simulink model "Motor_Model"  (Simulink 8.4)
settings: Solver=ode45  StartTime=0.0  StopTime=1  RelTol=1e-3
values from neighbouring files (symbols this model uses):
  eta = 0.9    [gs.m]
  g = 9.82    [gs.m]
  Ik = 0.004    [gs.m]
  Is = Ms*rs^2/2    (= 0.0005625)    [gs.m]
  J = 138E-7    (= 1.38e-05)    [gs.m]
  K_emf = 1/158    (= 0.00632911392405)    [gs.m]
  Kt = 60.3*10^-3    (= 0.0603)    [gs.m]
  l = 0.17    [gs.m]
  L = 0.329E-3    (= 0.000329)    [gs.m]
  max_current = 1    [gs.m]
  max_voltage = 48    [gs.m]
  Mtot = alu_mass + motor_mass + motor_power + arduino_mass + extra + M_s    (= 1.55)    [gs.m]
  Rm = 1.16    [gs.m]
settings Model: Creator=maen  LastModifiedBy=MikaelSjostedt
settings DataIOCC: LimitDataPoints=off

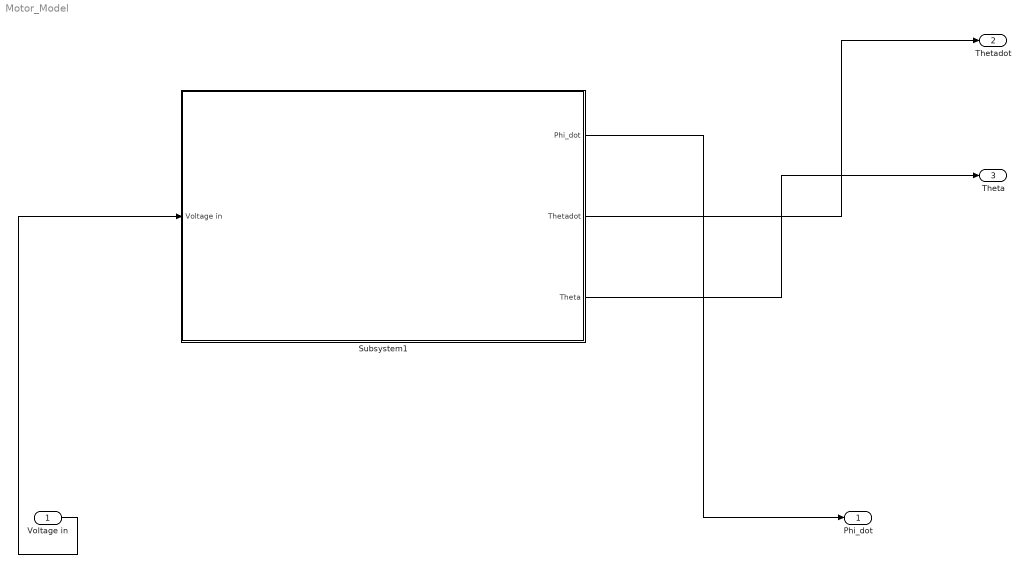
== system Motor_Model ==
  "Voltage in " : Inport
  Subsystem1 : Subsystem
  Phi_dot : Outport
  "Thetadot " : Outport  Port=2
  Theta : Outport  Port=3
  wires:
  "Voltage in "/1 -> Subsystem1/1("Voltage in ")
  Subsystem1/1(Phi_dot) -> Phi_dot/1
  Subsystem1/2("Thetadot ") -> "Thetadot "/1
  Subsystem1/3(Theta) -> Theta/1

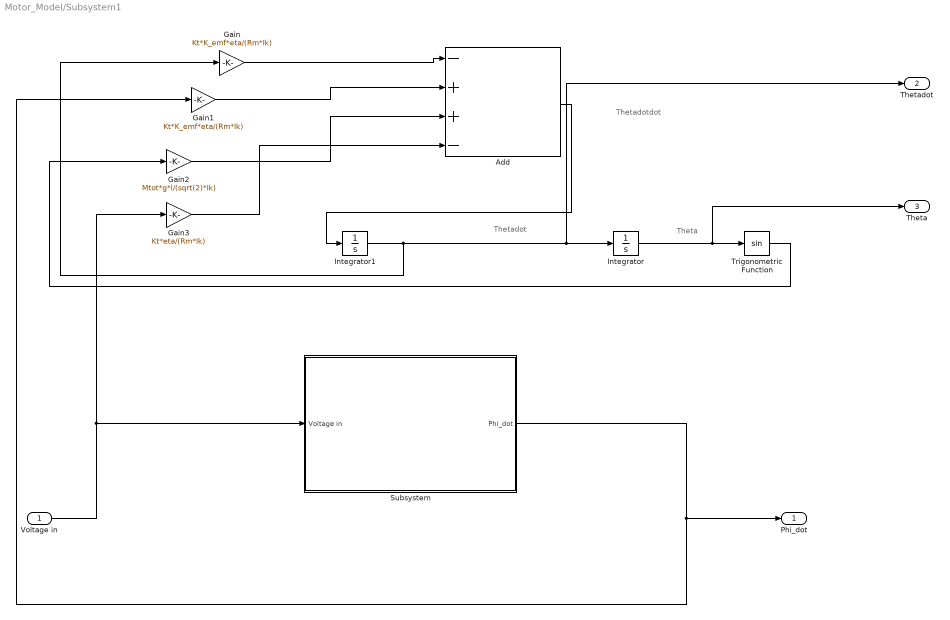
== system Motor_Model/Subsystem1 ==
  note: Theta
  note: Thetadot
  note: Thetadotdot
  "Voltage in " : Inport
  Add : Sum  Inputs=-++-
  Gain : Gain  Gain=Kt*K_emf*eta/(Rm*Ik)
  Gain1 : Gain  Gain=Kt*K_emf*eta/(Rm*Ik)
  Gain2 : Gain  Gain=Mtot*g*l/(sqrt(2)*Ik)
  Gain3 : Gain  Gain=Kt*eta/(Rm*Ik)
  Integrator : Integrator
  Integrator1 : Integrator
  Subsystem : Subsystem
  Trigonometric Function : Trigonometry
  Phi_dot : Outport
  "Thetadot " : Outport  Port=2
  Theta : Outport  Port=3
  wires:
  Trigonometric Function/1 -> Gain2/1
  Integrator/1 -> Theta/1, Trigonometric Function/1
  Integrator1/1 -> Gain/1, "Thetadot "/1, Integrator/1
  Add/1 -> Integrator1/1
  Gain3/1 -> Add/4
  Gain1/1 -> Add/2
  Gain/1 -> Add/1
  Gain2/1 -> Add/3
  Subsystem/1(Phi_dot) -> Phi_dot/1, Gain1/1
  "Voltage in "/1 -> Gain3/1, Subsystem/1("Voltage in ")

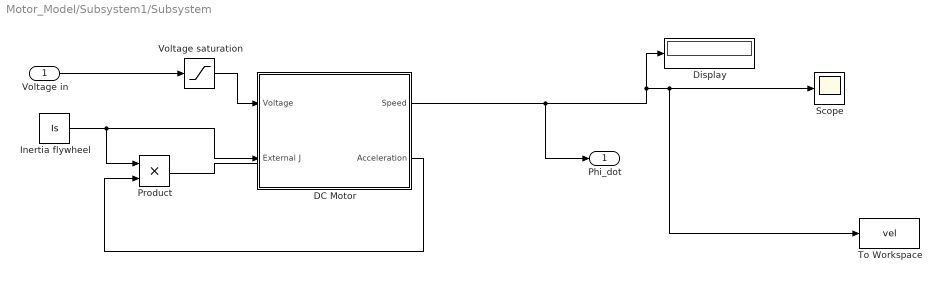
== system Motor_Model/Subsystem1/Subsystem ==
  "Voltage in " : Inport
  DC Motor : Subsystem
  Display : Display
  "Inertia flywheel " : Constant  Value=Is
  Product : Product
  Scope : Scope
  To Workspace : ToWorkspace  VariableName=vel  SampleTime=-1
  Voltage saturation : Saturate  UpperLimit=max_voltage  LowerLimit=-max_voltage
  Phi_dot : Outport
  wires:
  DC Motor/1(" Speed") -> Phi_dot/1, Display/1, To Workspace/1, Scope/1
  "Voltage in "/1 -> Voltage saturation/1
  Voltage saturation/1 -> DC Motor/1(Voltage)
  "Inertia flywheel "/1 -> Product/1, DC Motor/2(External J)
  DC Motor/2(Acceleration) -> Product/2
  Product/1 -> ?

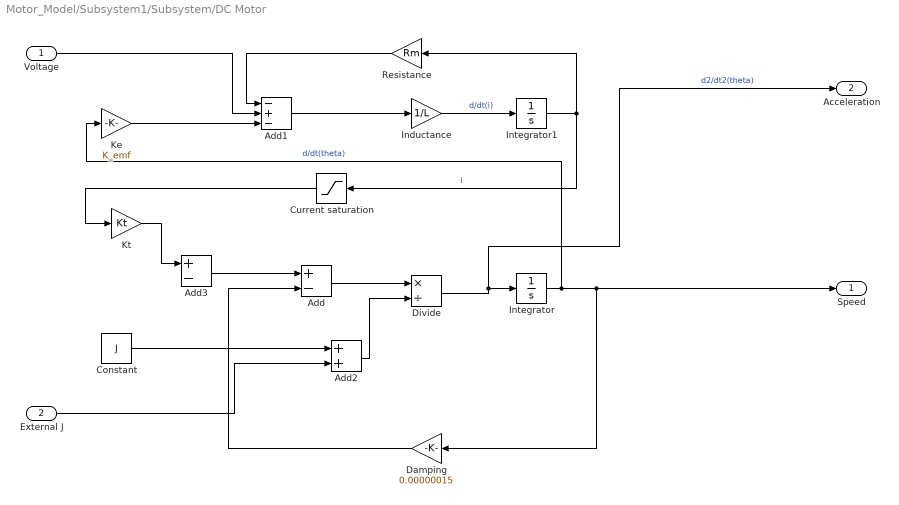
== system Motor_Model/Subsystem1/Subsystem/DC Motor ==
  Voltage : Inport
  External J : Inport  Port=2
  Add : Sum  Inputs=+-
  Add1 : Sum  Inputs=-+-
  Add2 : Sum
  Add3 : Sum  Inputs=+-
  Constant : Constant  Value=J
  Current saturation : Saturate  UpperLimit=max_current  LowerLimit=-max_current
  Damping : Gain  Gain=0.00000015
  Divide : Product  Inputs=*/
  Inductance : Gain  Gain=1/L
  Integrator : Integrator
  Integrator1 : Integrator
  Ke : Gain  Gain=K_emf
  Kt : Gain  Gain=Kt
  Resistance : Gain  Gain=Rm
  " Speed" : Outport
  Acceleration : Outport  Port=2
  wires:
  Integrator1/1 -> Current saturation/1, Resistance/1  "i"
  Inductance/1 -> Integrator1/1  "d/dt(i)"
  Divide/1 -> Acceleration/1, Integrator/1  "d2/dt2(theta)"
  Integrator/1 -> Ke/1, " Speed"/1, Damping/1  "d/dt(theta)"
  Add1/1 -> Inductance/1
  Add/1 -> Divide/1
  Damping/1 -> Add/2
  Kt/1 -> Add3/1
  Resistance/1 -> Add1/1
  Ke/1 -> Add1/3
  Voltage/1 -> Add1/2
  External J/1 -> Add2/2
  Constant/1 -> Add2/1
  Add2/1 -> Divide/2
  Current saturation/1 -> Kt/1
  Add3/1 -> Add/1
